simulink model "BD_SER2"  (Simulink 4.1.1)
settings: Solver=ode1  SolverMode=SingleTasking  StartTime=0.0  StopTime=max(cyc_mph(:,1))  FixedStep=1  MaxStep=1  RelTol=1e-3  AbsTol=1e-3
undefined symbols (not defined in the file): air_cp, amb_tmp, cyc_avg_time, cyc_cargo_mass, cyc_elevation_init, cyc_filter_bool, cyc_grade, cyc_mph, enable_stop, ess_cap_scale, ess_coulombic_eff, ess_init_soc, ess_max_ah_cap, ess_max_volts, ess_min_volts, ess_mod_airflow, ess_mod_cp, ess_mod_init_tmp, ess_module_mass, ess_module_num, ess_on, ess_res_scale_coef, ess_res_scale_fun, ess_set_tmp, ess_th_calc, ess_th_res_off, ess_th_res_on, ess_tmp, ess_voc, ex_calc, fc_ct_trq, fc_emis, fc_inertia, fc_map_spd, fc_max_trq, fc_spd_scale, fc_trq_scale, fd_inertia, fd_loss, fd_ratio, gb_dnshift_load, gb_dnshift_spd, gb_gears_num, gb_inertia, gb_num_init, gb_ratio, gb_shift_delay, gb_spd_scale, gb_trq_scale, gb_upshift_load, gb_upshift_spd, gc_inertia, gc_map_spd, gc_map_trq, gc_max_crrnt, gc_max_trq, gc_outpwr_map, gc_overtrq_factor, gc_spd_scale, gc_trq_scale ... (+37)
libraries: lib_wheel2 x12, lib_accessory2 x4, lib_controls2 x3, lib_etc x2, lib_help x2, lib_fuel_converter x2, lib_drive_cycle2 x1, lib_interactive x1, lib_drive_cycle x1, lib_exhaust x1, lib_fuel_converter3 x1
(part 3 of 15)

== system BD_SER2/ACC ELEC <acce>/ACC ELEC model and interface/electrical accessory model ==
  note: Backward-Forward Models
  "requested electrical Power, out to the driveline (W)" : Inport  Port=1  LatchInput=off
  achieved power in from power source (W) : Inport  Port=2  LatchInput=off
  Block NOTES : Subsystem
      settings: RTWFcnNameOpts=Auto  RTWFileNameOpts=Auto
      mask Display: disp('Block\nNOTES')
  backward model : Subsystem
      settings: RTWFcnNameOpts=Auto  RTWFileNameOpts=Auto
  electrical power logging : lib_accessory2/SubLibraries/electrical power logging  eff=acc_mech_eff
      link override enhancedToWorkspace1/To Workspace: VariableName=acce_elec_pwr_in_a  SampleTime=-1  SaveFormat=Array
  enhancedToWorkspace : Subsystem  TreatAsAtomicUnit=on  mask(enhancedToWorkspace){generalName=generalName, specificName=elec_pwr_a, logFlag=logFlag}
      mask prompts: generalName "General Name [char-evaluated]"; specificName "Specific Name [char-literal]"; logFlag "Enable flag (1=on,0=off)"
      mask help: A wrapper for the Simulink "To Workspace" block that allows you to evaluate the name of the variable to log to workspace. This is useful to avoid the double logging errors that occur when you pull in two library models that attempt to log to the same variable.
      mask init:
      | enhancedToWsMaker
      settings: CopyFcn=breakLinkCopyFcn  ParentCloseFcn=breakLinkParCloseFcn  RTWFcnNameOpts=Auto  RTWFileNameOpts=Auto
      mask Help:
      | <h2>Enhanced To Workspace Block</h2>
      | <h3>Parameters</h3>
      | <UL>
      | <li><b>General Name:</b> This is the more general name of the variable. Variables are saved to the workspace as <i>generalName_specificName</i>. Note that this is an evaluated variable. If you would like to type in the value directly, it must be surrounded with single quotes. Otherwise you can input the name of a variable containing a char string.</li>
      | <li><b>Specific Name:</b> This is the specific name of the variable. Note that this is input as a char literal (i.e., you don't need quotes).</li>
      | <li><b>Enable Flag:</b> This flag should have the value of 0 or 1. If 0, the variable will not be logged to the workspace. If 1, the variable will be logged. This is done so that variable logging can be turned off to improve speed.</li>
      | </ul>
      | <h3>Overview</h3>
      | <p>The enhanced to workspace block was put together to allow one to dynamically resolve variable names at run time in simulink. This is most powerful when used in conjunction with a masked subsystem to allow multiple instances of that masked subsytem to be used in the same model. The strategy is to set the generalName in the block mask which will allow the block to change the general name for all variable logging on the fly.
      | <h3>Helper Files</h3>
      | <p>Three m-files are required by the enhancedToWorkspace block. These files are located in the &lt; ADVISOR root &gt;/GUI directory :
      | <ul>
      | <li><i>enhancedToWsMaker.m</i> This file runs the mask initialization for the block</li>
      | <li><i>breakLinkCopyFcn.m</i> This file is used by the block callback when the simulink block is copied. It is necessary to break the link to the enhancedToWorkspace similar to the To Workspace block in order for it to be able to configure itself. (Try copying simulink's To Workspace block--it is impossible to make a link)</li>
      | <li><i>breakLinkParCloseFcn.m</i> This file is similar to the breakLinkCopyFcn and is used when a parent system is closed</li>
      | </ul>
      | <hr>
      | 
      | <p>Created 2003-Jan-21, Michael Patrick O'Keefe, NREL</p>
      | 
      | <!--
      | <VARDEF>
      | <H3>var_name</H3>
      | <UL>
      | <LI><B>data type</B> data type here</LI>
      | <LI><B>units</B> units here</LI>
      | <LI><B>vehicle type</B> vehicle type here</LI>
      | <LI><B>description</B> description here</LI>
      | </UL>
      | </VARDEF>
      | -->
      mask Display: disp([generalName,'_',specificName])
  enhancedToWorkspace1 : Subsystem  TreatAsAtomicUnit=on  mask(enhancedToWorkspace){generalName=generalName, specificName=elec_pwr_r, logFlag=logFlag}
      mask prompts: generalName "General Name [char-evaluated]"; specificName "Specific Name [char-literal]"; logFlag "Enable flag (1=on,0=off)"
      mask help: A wrapper for the Simulink "To Workspace" block that allows you to evaluate the name of the variable to log to workspace. This is useful to avoid the double logging errors that occur when you pull in two library models that attempt to log to the same variable.
      mask init:
      | enhancedToWsMaker
      settings: CopyFcn=breakLinkCopyFcn  ParentCloseFcn=breakLinkParCloseFcn  RTWFcnNameOpts=Auto  RTWFileNameOpts=Auto
      mask Help:
      | <h2>Enhanced To Workspace Block</h2>
      | <h3>Parameters</h3>
      | <UL>
      | <li><b>General Name:</b> This is the more general name of the variable. Variables are saved to the workspace as <i>generalName_specificName</i>. Note that this is an evaluated variable. If you would like to type in the value directly, it must be surrounded with single quotes. Otherwise you can input the name of a variable containing a char string.</li>
      | <li><b>Specific Name:</b> This is the specific name of the variable. Note that this is input as a char literal (i.e., you don't need quotes).</li>
      | <li><b>Enable Flag:</b> This flag should have the value of 0 or 1. If 0, the variable will not be logged to the workspace. If 1, the variable will be logged. This is done so that variable logging can be turned off to improve speed.</li>
      | </ul>
      | <h3>Overview</h3>
      | <p>The enhanced to workspace block was put together to allow one to dynamically resolve variable names at run time in simulink. This is most powerful when used in conjunction with a masked subsystem to allow multiple instances of that masked subsytem to be used in the same model. The strategy is to set the generalName in the block mask which will allow the block to change the general name for all variable logging on the fly.
      | <h3>Helper Files</h3>
      | <p>Three m-files are required by the enhancedToWorkspace block. These files are located in the &lt; ADVISOR root &gt;/GUI directory :
      | <ul>
      | <li><i>enhancedToWsMaker.m</i> This file runs the mask initialization for the block</li>
      | <li><i>breakLinkCopyFcn.m</i> This file is used by the block callback when the simulink block is copied. It is necessary to break the link to the enhancedToWorkspace similar to the To Workspace block in order for it to be able to configure itself. (Try copying simulink's To Workspace block--it is impossible to make a link)</li>
      | <li><i>breakLinkParCloseFcn.m</i> This file is similar to the breakLinkCopyFcn and is used when a parent system is closed</li>
      | </ul>
      | <hr>
      | 
      | <p>Created 2003-Jan-21, Michael Patrick O'Keefe, NREL</p>
      | 
      | <!--
      | <VARDEF>
      | <H3>var_name</H3>
      | <UL>
      | <LI><B>data type</B> data type here</LI>
      | <LI><B>units</B> units here</LI>
      | <LI><B>vehicle type</B> vehicle type here</LI>
      | <LI><B>description</B> description here</LI>
      | </UL>
      | </VARDEF>
      | -->
      mask Display: disp([generalName,'_',specificName])
  forward model : Subsystem
      settings: RTWFcnNameOpts=Auto  RTWFileNameOpts=Auto
  "requested electrical Power, in from the power source (W)" : Outport  Port=1
  "achieved electrical Power, out to the driveline (W)" : Outport  Port=2
  tag scope: acc_elec_pwr_a=scoped, acc_elec_pwr_r=scoped
  wires:
  forward model/2(acc_pwr_out) -> electrical power logging/1, enhancedToWorkspace/1(In1), [acc_elec_pwr_a]
  backward model/2(elec_acc_out) -> enhancedToWorkspace1/1(In1), forward model/2(acc_pwr_in), [acc_elec_pwr_r]
  forward model/1(pwr_out) -> "achieved electrical Power, out to the driveline (W)"/1
  achieved power in from power source (W)/1 -> forward model/1(pwr_in)
  backward model/1(elec_out) -> "requested electrical Power, in from the power source (W)"/1
  "requested electrical Power, out to the driveline (W)"/1 -> backward model/1(pwr_in)

== system BD_SER2/ACC ELEC <acce>/ACC ELEC model and interface/signal annotator ==
  In1 : Inport  Port=1  LatchInput=off
  Out1 : Outport  Port=1
  wires:
  In1/1 -> Out1/1  "driveline_elec_pwr_r"

== system BD_SER2/ACC MECH <accm>/mechanical accessory model and interface/Block NOTES ==

== system BD_SER2/ACC MECH <accm>/mechanical accessory model and interface/Mechanical Accessory model ==
  note: Reference Speed for speed dependant accessories
  note: Backward-Forward Models
  "requested shaft T and w, out to the driveline  (Nm ; rad/s; rad/s)" : Inport  Port=1  LatchInput=off
  "achieved shaft and belt T and w, in from the prime mover (Nm ; rad/s)" : Inport  Port=2  LatchInput=off
  Block NOTES : Subsystem
      settings: RTWFcnNameOpts=Auto  RTWFileNameOpts=Auto
      mask Display: disp('Block\nNOTES')
  Demux : Demux  Outputs=2  BusSelectionMode=off
  Demux1 : Demux  Outputs=2  BusSelectionMode=off
  Mux1 : Mux  Inputs=2
  Mux2 : Mux  Inputs=2
  backward model : Subsystem
      settings: RTWFcnNameOpts=Auto  RTWFileNameOpts=Auto
  f1 : Subsystem  TreatAsAtomicUnit=on  mask(enhancedToWorkspace){generalName=generalName, specificName=mech_pwr_a, logFlag=logFlag}
      mask prompts: generalName "General Name [char-evaluated]"; specificName "Specific Name [char-literal]"; logFlag "Enable flag (1=on,0=off)"
      mask help: A wrapper for the Simulink "To Workspace" block that allows you to evaluate the name of the variable to log to workspace. This is useful to avoid the double logging errors that occur when you pull in two library models that attempt to log to the same variable.
      mask init:
      | enhancedToWsMaker
      settings: CopyFcn=breakLinkCopyFcn  ParentCloseFcn=breakLinkParCloseFcn  RTWFcnNameOpts=Auto  RTWFileNameOpts=Auto
      mask Help:
      | <h2>Enhanced To Workspace Block</h2>
      | <h3>Parameters</h3>
      | <UL>
      | <li><b>General Name:</b> This is the more general name of the variable. Variables are saved to the workspace as <i>generalName_specificName</i>. Note that this is an evaluated variable. If you would like to type in the value directly, it must be surrounded with single quotes. Otherwise you can input the name of a variable containing a char string.</li>
      | <li><b>Specific Name:</b> This is the specific name of the variable. Note that this is input as a char literal (i.e., you don't need quotes).</li>
      | <li><b>Enable Flag:</b> This flag should have the value of 0 or 1. If 0, the variable will not be logged to the workspace. If 1, the variable will be logged. This is done so that variable logging can be turned off to improve speed.</li>
      | </ul>
      | <h3>Overview</h3>
      | <p>The enhanced to workspace block was put together to allow one to dynamically resolve variable names at run time in simulink. This is most powerful when used in conjunction with a masked subsystem to allow multiple instances of that masked subsytem to be used in the same model. The strategy is to set the generalName in the block mask which will allow the block to change the general name for all variable logging on the fly.
      | <h3>Helper Files</h3>
      | <p>Three m-files are required by the enhancedToWorkspace block. These files are located in the &lt; ADVISOR root &gt;/GUI directory :
      | <ul>
      | <li><i>enhancedToWsMaker.m</i> This file runs the mask initialization for the block</li>
      | <li><i>breakLinkCopyFcn.m</i> This file is used by the block callback when the simulink block is copied. It is necessary to break the link to the enhancedToWorkspace similar to the To Workspace block in order for it to be able to configure itself. (Try copying simulink's To Workspace block--it is impossible to make a link)</li>
      | <li><i>breakLinkParCloseFcn.m</i> This file is similar to the breakLinkCopyFcn and is used when a parent system is closed</li>
      | </ul>
      | <hr>
      | 
      | <p>Created 2003-Jan-21, Michael Patrick O'Keefe, NREL</p>
      | 
      | <!--
      | <VARDEF>
      | <H3>var_name</H3>
      | <UL>
      | <LI><B>data type</B> data type here</LI>
      | <LI><B>units</B> units here</LI>
      | <LI><B>vehicle type</B> vehicle type here</LI>
      | <LI><B>description</B> description here</LI>
      | </UL>
      | </VARDEF>
      | -->
      mask Display: disp([generalName,'_',specificName])
  f2 : Subsystem  TreatAsAtomicUnit=on  mask(enhancedToWorkspace){generalName=generalName, specificName=mech_trq_a, logFlag=logFlag}
      mask prompts: generalName "General Name [char-evaluated]"; specificName "Specific Name [char-literal]"; logFlag "Enable flag (1=on,0=off)"
      mask help: A wrapper for the Simulink "To Workspace" block that allows you to evaluate the name of the variable to log to workspace. This is useful to avoid the double logging errors that occur when you pull in two library models that attempt to log to the same variable.
      mask init:
      | enhancedToWsMaker
      settings: CopyFcn=breakLinkCopyFcn  ParentCloseFcn=breakLinkParCloseFcn  RTWFcnNameOpts=Auto  RTWFileNameOpts=Auto
      mask Help:
      | <h2>Enhanced To Workspace Block</h2>
      | <h3>Parameters</h3>
      | <UL>
      | <li><b>General Name:</b> This is the more general name of the variable. Variables are saved to the workspace as <i>generalName_specificName</i>. Note that this is an evaluated variable. If you would like to type in the value directly, it must be surrounded with single quotes. Otherwise you can input the name of a variable containing a char string.</li>
      | <li><b>Specific Name:</b> This is the specific name of the variable. Note that this is input as a char literal (i.e., you don't need quotes).</li>
      | <li><b>Enable Flag:</b> This flag should have the value of 0 or 1. If 0, the variable will not be logged to the workspace. If 1, the variable will be logged. This is done so that variable logging can be turned off to improve speed.</li>
      | </ul>
      | <h3>Overview</h3>
      | <p>The enhanced to workspace block was put together to allow one to dynamically resolve variable names at run time in simulink. This is most powerful when used in conjunction with a masked subsystem to allow multiple instances of that masked subsytem to be used in the same model. The strategy is to set the generalName in the block mask which will allow the block to change the general name for all variable logging on the fly.
      | <h3>Helper Files</h3>
      | <p>Three m-files are required by the enhancedToWorkspace block. These files are located in the &lt; ADVISOR root &gt;/GUI directory :
      | <ul>
      | <li><i>enhancedToWsMaker.m</i> This file runs the mask initialization for the block</li>
      | <li><i>breakLinkCopyFcn.m</i> This file is used by the block callback when the simulink block is copied. It is necessary to break the link to the enhancedToWorkspace similar to the To Workspace block in order for it to be able to configure itself. (Try copying simulink's To Workspace block--it is impossible to make a link)</li>
      | <li><i>breakLinkParCloseFcn.m</i> This file is similar to the breakLinkCopyFcn and is used when a parent system is closed</li>
      | </ul>
      | <hr>
      | 
      | <p>Created 2003-Jan-21, Michael Patrick O'Keefe, NREL</p>
      | 
      | <!--
      | <VARDEF>
      | <H3>var_name</H3>
      | <UL>
      | <LI><B>data type</B> data type here</LI>
      | <LI><B>units</B> units here</LI>
      | <LI><B>vehicle type</B> vehicle type here</LI>
      | <LI><B>description</B> description here</LI>
      | </UL>
      | </VARDEF>
      | -->
      mask Display: disp([generalName,'_',specificName])
  forward model : Subsystem
      settings: RTWFcnNameOpts=Auto  RTWFileNameOpts=Auto
  limit accessory mechanical speed achieved : lib_etc/saturation with inputs
      settings: RTWFcnNameOpts=Auto  RTWFileNameOpts=Auto
  limit accessory mechanical speed request : lib_etc/saturation with inputs
      settings: RTWFcnNameOpts=Auto  RTWFileNameOpts=Auto
  mechanical power logging : lib_accessory2/SubLibraries/mechanical power logging  eff=acc_mech_eff
  "requested shaft and belt T and w, in from the prime mover (Nm ; rad/s)" : Outport  Port=1
  "achieved shaft T and w, out to the driveline (Nm ; rad/s)" : Outport  Port=2
  tag scope: acc_mech_pwr_a=scoped, acc_mech_trq_a=scoped, w_APU_speed=scoped
  wires:
  [acc_min_spd] -> limit accessory mechanical speed achieved/3
  [acc_max_spd] -> limit accessory mechanical speed achieved/1
  [acc_mech_spd_a] -> limit accessory mechanical speed achieved/2
  limit accessory mechanical speed achieved/1 -> forward model/2(spd_in)
  [acc_min_spd] -> limit accessory mechanical speed request/3
  [acc_max_spd] -> limit accessory mechanical speed request/1
  limit accessory mechanical speed request/1 -> [w_APU_speed], backward model/2(spd_in)
  [acc_mech_spd_r] -> limit accessory mechanical speed request/2
  [acc_mech_trq_r] -> forward model/3(acc_trq_req)
  forward model/3(acc_mech_pwr_a) -> mechanical power logging/1, f1/1(In1), [acc_mech_pwr_a]
  forward model/2(acc_mech_trq_a) -> f2/1(In1), [acc_mech_trq_a]
  Mux2/1 -> "achieved shaft T and w, out to the driveline (Nm ; rad/s)"/1
  Mux1/1 -> "requested shaft and belt T and w, in from the prime mover (Nm ; rad/s)"/1
  "achieved shaft and belt T and w, in from the prime mover (Nm ; rad/s)"/1 -> Demux1/1
  "requested shaft T and w, out to the driveline  (Nm ; rad/s; rad/s)"/1 -> Demux/1
  Demux/1 -> backward model/1(trq1)  "trq out r"
  Demux/2 -> Mux1/2  "w shaft out r"
  backward model/1(trq2) -> Mux1/1  "trq in r"
  forward model/1(trq_out) -> Mux2/1
  Demux1/1 -> forward model/1(trq_in)  "trq in achieved from prime mover"
  Demux1/2 -> Mux2/2  "w shaft achieved by prime mover"

== system BD_SER2/ACC MECH <accm>/mechanical accessory model and interface/help ==

== system BD_SER2/ACC MECH <accm>/mechanical accessory model and interface/signal annotator ==
  In1 : Inport  Port=1  LatchInput=off
  Demux : Demux  Outputs=2  BusSelectionMode=off
  Mux : Mux  Inputs=2
  enhancedToWorkspace : Subsystem  TreatAsAtomicUnit=on  mask(enhancedToWorkspace){generalName=generalName, specificName=pre_acc_spd_out_r, logFlag=logFlag}
      mask prompts: generalName "General Name [char-evaluated]"; specificName "Specific Name [char-literal]"; logFlag "Enable flag (1=on,0=off)"
      mask help: A wrapper for the Simulink "To Workspace" block that allows you to evaluate the name of the variable to log to workspace. This is useful to avoid the double logging errors that occur when you pull in two library models that attempt to log to the same variable.
      mask init:
      | enhancedToWsMaker
      settings: CopyFcn=breakLinkCopyFcn  ParentCloseFcn=breakLinkParCloseFcn  RTWFcnNameOpts=Auto  RTWFileNameOpts=Auto
      mask Help:
      | <h2>Enhanced To Workspace Block</h2>
      | <h3>Parameters</h3>
      | <UL>
      | <li><b>General Name:</b> This is the more general name of the variable. Variables are saved to the workspace as <i>generalName_specificName</i>. Note that this is an evaluated variable. If you would like to type in the value directly, it must be surrounded with single quotes. Otherwise you can input the name of a variable containing a char string.</li>
      | <li><b>Specific Name:</b> This is the specific name of the variable. Note that this is input as a char literal (i.e., you don't need quotes).</li>
      | <li><b>Enable Flag:</b> This flag should have the value of 0 or 1. If 0, the variable will not be logged to the workspace. If 1, the variable will be logged. This is done so that variable logging can be turned off to improve speed.</li>
      | </ul>
      | <h3>Overview</h3>
      | <p>The enhanced to workspace block was put together to allow one to dynamically resolve variable names at run time in simulink. This is most powerful when used in conjunction with a masked subsystem to allow multiple instances of that masked subsytem to be used in the same model. The strategy is to set the generalName in the block mask which will allow the block to change the general name for all variable logging on the fly.
      | <h3>Helper Files</h3>
      | <p>Three m-files are required by the enhancedToWorkspace block. These files are located in the &lt; ADVISOR root &gt;/GUI directory :
      | <ul>
      | <li><i>enhancedToWsMaker.m</i> This file runs the mask initialization for the block</li>
      | <li><i>breakLinkCopyFcn.m</i> This file is used by the block callback when the simulink block is copied. It is necessary to break the link to the enhancedToWorkspace similar to the To Workspace block in order for it to be able to configure itself. (Try copying simulink's To Workspace block--it is impossible to make a link)</li>
      | <li><i>breakLinkParCloseFcn.m</i> This file is similar to the breakLinkCopyFcn and is used when a parent system is closed</li>
      | </ul>
      | <hr>
      | 
      | <p>Created 2003-Jan-21, Michael Patrick O'Keefe, NREL</p>
      | 
      | <!--
      | <VARDEF>
      | <H3>var_name</H3>
      | <UL>
      | <LI><B>data type</B> data type here</LI>
      | <LI><B>units</B> units here</LI>
      | <LI><B>vehicle type</B> vehicle type here</LI>
      | <LI><B>description</B> description here</LI>
      | </UL>
      | </VARDEF>
      | -->
      mask Display: disp([generalName,'_',specificName])
  enhancedToWorkspace1 : Subsystem  TreatAsAtomicUnit=on  mask(enhancedToWorkspace){generalName=generalName, specificName=pre_acc_trq_out_r, logFlag=logFlag}
      mask prompts: generalName "General Name [char-evaluated]"; specificName "Specific Name [char-literal]"; logFlag "Enable flag (1=on,0=off)"
      mask help: A wrapper for the Simulink "To Workspace" block that allows you to evaluate the name of the variable to log to workspace. This is useful to avoid the double logging errors that occur when you pull in two library models that attempt to log to the same variable.
      mask init:
      | enhancedToWsMaker
      settings: CopyFcn=breakLinkCopyFcn  ParentCloseFcn=breakLinkParCloseFcn  RTWFcnNameOpts=Auto  RTWFileNameOpts=Auto
      mask Help:
      | <h2>Enhanced To Workspace Block</h2>
      | <h3>Parameters</h3>
      | <UL>
      | <li><b>General Name:</b> This is the more general name of the variable. Variables are saved to the workspace as <i>generalName_specificName</i>. Note that this is an evaluated variable. If you would like to type in the value directly, it must be surrounded with single quotes. Otherwise you can input the name of a variable containing a char string.</li>
      | <li><b>Specific Name:</b> This is the specific name of the variable. Note that this is input as a char literal (i.e., you don't need quotes).</li>
      | <li><b>Enable Flag:</b> This flag should have the value of 0 or 1. If 0, the variable will not be logged to the workspace. If 1, the variable will be logged. This is done so that variable logging can be turned off to improve speed.</li>
      | </ul>
      | <h3>Overview</h3>
      | <p>The enhanced to workspace block was put together to allow one to dynamically resolve variable names at run time in simulink. This is most powerful when used in conjunction with a masked subsystem to allow multiple instances of that masked subsytem to be used in the same model. The strategy is to set the generalName in the block mask which will allow the block to change the general name for all variable logging on the fly.
      | <h3>Helper Files</h3>
      | <p>Three m-files are required by the enhancedToWorkspace block. These files are located in the &lt; ADVISOR root &gt;/GUI directory :
      | <ul>
      | <li><i>enhancedToWsMaker.m</i> This file runs the mask initialization for the block</li>
      | <li><i>breakLinkCopyFcn.m</i> This file is used by the block callback when the simulink block is copied. It is necessary to break the link to the enhancedToWorkspace similar to the To Workspace block in order for it to be able to configure itself. (Try copying simulink's To Workspace block--it is impossible to make a link)</li>
      | <li><i>breakLinkParCloseFcn.m</i> This file is similar to the breakLinkCopyFcn and is used when a parent system is closed</li>
      | </ul>
      | <hr>
      | 
      | <p>Created 2003-Jan-21, Michael Patrick O'Keefe, NREL</p>
      | 
      | <!--
      | <VARDEF>
      | <H3>var_name</H3>
      | <UL>
      | <LI><B>data type</B> data type here</LI>
      | <LI><B>units</B> units here</LI>
      | <LI><B>vehicle type</B> vehicle type here</LI>
      | <LI><B>description</B> description here</LI>
      | </UL>
      | </VARDEF>
      | -->
      mask Display: disp([generalName,'_',specificName])
  Out1 : Outport  Port=1
  wires:
  Mux/1 -> Out1/1
  Demux/2 -> Mux/2, enhancedToWorkspace/1(In1)  "macc_spd_out_r"
  Demux/1 -> Mux/1, enhancedToWorkspace1/1(In1)  "macc_trq_out_r"
  In1/1 -> Demux/1

== system BD_SER2/drive cycle <cyc>/drive cycle model and interface/drive cycle model ==
  Backlash : Backlash  BacklashWidth=0.5  InitialOutput=0
  Block NOTES : Subsystem
      settings: RTWFcnNameOpts=Auto  RTWFileNameOpts=Auto
      mask Display: disp('Block\nNOTES')
  Constant : Constant  Value=0.001
  Constant1 : Constant  Orientation=left  Value=0
  Constant2 : Constant  Value=cyc_filter_bool
  Derivative : Derivative
  Integrator : Integrator  ExternalReset=none  InitialConditionSource=internal  InitialCondition=cyc_elevation_init  LimitOutput=off  UpperSaturationLimit=inf  LowerSaturationLimit=-inf  ShowSaturationPort=off  ShowStatePort=off  AbsoluteTolerance=auto
  Product : Product  Inputs=2  Multiplication=Element-wise(.*)  SaturateOnIntegerOverflow=on
  Relational Operator : RelationalOperator  Operator=>
  Switch : Switch  Threshold=eps
  Switch1 : Switch  Threshold=eps
  Switch2 : Switch  Threshold=1
  Switch3 : Switch  Threshold=1
  Trigonometric Function : Trigonometry  Operator=sin  OutputSignalType=auto
  distance travelled (m) : Subsystem
      settings: RTWFcnNameOpts=Auto  RTWFileNameOpts=Auto
  enhancedToWorkspace : Subsystem  TreatAsAtomicUnit=on  mask(enhancedToWorkspace){generalName=generalName, specificName=cargo_mass_vs_time, logFlag=logFlag}
      mask prompts: generalName "General Name [char-evaluated]"; specificName "Specific Name [char-literal]"; logFlag "Enable flag (1=on,0=off)"
      mask help: A wrapper for the Simulink "To Workspace" block that allows you to evaluate the name of the variable to log to workspace. This is useful to avoid the double logging errors that occur when you pull in two library models that attempt to log to the same variable.
      mask init:
      | enhancedToWsMaker
      settings: CopyFcn=breakLinkCopyFcn  ParentCloseFcn=breakLinkParCloseFcn  RTWFcnNameOpts=Auto  RTWFileNameOpts=Auto
      mask Help:
      | <h2>Enhanced To Workspace Block</h2>
      | <h3>Parameters</h3>
      | <UL>
      | <li><b>General Name:</b> This is the more general name of the variable. Variables are saved to the workspace as <i>generalName_specificName</i>. Note that this is an evaluated variable. If you would like to type in the value directly, it must be surrounded with single quotes. Otherwise you can input the name of a variable containing a char string.</li>
      | <li><b>Specific Name:</b> This is the specific name of the variable. Note that this is input as a char literal (i.e., you don't need quotes).</li>
      | <li><b>Enable Flag:</b> This flag should have the value of 0 or 1. If 0, the variable will not be logged to the workspace. If 1, the variable will be logged. This is done so that variable logging can be turned off to improve speed.</li>
      | </ul>
      | <h3>Overview</h3>
      | <p>The enhanced to workspace block was put together to allow one to dynamically resolve variable names at run time in simulink. This is most powerful when used in conjunction with a masked subsystem to allow multiple instances of that masked subsytem to be used in the same model. The strategy is to set the generalName in the block mask which will allow the block to change the general name for all variable logging on the fly.
      | <h3>Helper Files</h3>
      | <p>Three m-files are required by the enhancedToWorkspace block. These files are located in the &lt; ADVISOR root &gt;/GUI directory :
      | <ul>
      | <li><i>enhancedToWsMaker.m</i> This file runs the mask initialization for the block</li>
      | <li><i>breakLinkCopyFcn.m</i> This file is used by the block callback when the simulink block is copied. It is necessary to break the link to the enhancedToWorkspace similar to the To Workspace block in order for it to be able to configure itself. (Try copying simulink's To Workspace block--it is impossible to make a link)</li>
      | <li><i>breakLinkParCloseFcn.m</i> This file is similar to the breakLinkCopyFcn and is used when a parent system is closed</li>
      | </ul>
      | <hr>
      | 
      | <p>Created 2003-Jan-21, Michael Patrick O'Keefe, NREL</p>
      | 
      | <!--
      | <VARDEF>
      | <H3>var_name</H3>
      | <UL>
      | <LI><B>data type</B> data type here</LI>
      | <LI><B>units</B> units here</LI>
      | <LI><B>vehicle type</B> vehicle type here</LI>
      | <LI><B>description</B> description here</LI>
      | </UL>
      | </VARDEF>
      | -->
      mask Display: disp([generalName,'_',specificName])
  mph-->m/s : Gain  Gain=0.447  Multiplication=Element-wise(K.*u)  SaturateOnIntegerOverflow=on
  repeated cycle grade vs. distance : Subsystem  mask(Repeating table){t=cyc_grade(:,1), y=cyc_grade(:,2)}
      mask prompts: t "Input values:"; y "Output values:"
      mask help:
      | Repeating table.
      | Enter values of input and output for first cycle.
      mask init:
      | period = max(@1);
      settings: RTWFcnNameOpts=Auto  RTWFileNameOpts=Auto
      mask Help: Repeats cycle given in table. Input values should be monotonically increasing.
  repeated cycle speed vs. time : Subsystem  mask(Repeating table){@1=cyc_mph(:,1), @2=cyc_mph(:,2)}
      mask prompts: @1 "Time values:"; @2 "Output values:"
      mask help:
      | Repeating table.
      | Enter values of time and output for first cycle.
      mask init:
      | period = max(@1); t = @1; y = @2;
      settings: RTWFcnNameOpts=Auto  RTWFileNameOpts=Auto
      mask Help: Repeats cycle given in table. Time values should be monotonically increasing.
  repeated cycle vehicle cargo mass vs. distance : lib_drive_cycle/drive cycle <cyc>/repeated cycle grade vs. distance  t=cyc_cargo_mass(:,1)  y=cyc_cargo_mass(:,2)
  "super-smooth, no-lag trace" : Subsystem  mask(Smooth Cycle){t=cyc_mph(:,1), y=cyc_mph(:,2), avgtime=cyc_avg_time}
      mask prompts: t "Time vector for trace (s):"; y "Speed vector for trace (km/hr):"; avgtime "Averaging time (s):"
      mask help: Smooth Cycle
      mask init:
      | period = max(@1);,
      settings: RTWFcnNameOpts=Auto  RTWFileNameOpts=Auto
      mask Display: disp('SMOOTH\nCYCLE')
  req'd vehicle speed (m/s) : Outport  Port=1  InitialOutput=0
  tag scope: cyc_mph_r=scoped, cyc_mph_r_orig=scoped, distance=scoped, elevation=scoped, grade=scoped, grade_orig=scoped, veh_cargo_mass=scoped
  wires:
  repeated cycle vehicle cargo mass vs. distance/1 -> enhancedToWorkspace/1(In1), [veh_cargo_mass]
  [Altia_Run] -> Switch3/2
  [altia_grade] -> Switch3/1
  [Altia_Run] -> Switch2/2
  [altia_cyc_mph_r] -> Switch2/1
  mph-->m/s/1 -> req'd vehicle speed (m/s)/1
  Switch2/1 -> mph-->m/s/1, [cyc_mph_r]
  Constant2/1 -> Switch1/2
  Constant1/1 -> Switch/3
  Relational Operator/1 -> Switch/2
  Backlash/1 -> Switch/1
  Constant/1 -> Relational Operator/2
  "super-smooth, no-lag trace"/1(out_1) -> Relational Operator/1, Backlash/1
  Switch/1 -> Switch1/1
  repeated cycle speed vs. time/1(out_1) -> Switch1/3
  Switch1/1 -> [cyc_mph_r_orig], Switch2/3
  Product/1 -> Integrator/1
  Derivative/1 -> Product/1
  Trigonometric Function/1 -> Product/2
  Integrator/1 -> [elevation]
  Switch3/1 -> [grade], Trigonometric Function/1
  distance travelled (m)/1(Out1) -> repeated cycle vehicle cargo mass vs. distance/1, [distance], Derivative/1, repeated cycle grade vs. distance/1(distance travelled (m))
  repeated cycle grade vs. distance/1(out_1) -> Switch3/3, [grade_orig]

== system BD_SER2/drive cycle <cyc>/drive cycle model and interface/signal annotator ==
  note: initial speed in m/s
  In1 : Inport  Port=1  LatchInput=off
  In2 : Inport  Port=2  LatchInput=off
  In3 : Inport  Port=3  LatchInput=off
  Bus Creator : BusCreator  Inputs=4
  Constant : Constant  Value=cyc_mph(1,2)*.447
  Out1 : Outport  Port=1
  wires:
  Constant/1 -> Bus Creator/4  "v_init"
  In3/1 -> Bus Creator/3  "cycle_mph_r"
  In2/1 -> Bus Creator/2  "cycle_mph_r_orig"
  Bus Creator/1 -> Out1/1
  In1/1 -> Bus Creator/1  "simulation_time"

== system BD_SER2/ess config/energy storage <ess>/Block NOTES ==
  note: This is a stand-alone version of an energy storage system
      |
      | Several different models are available

== system BD_SER2/ess config/energy storage <ess>/documentation9 ==

== system BD_SER2/ess config/energy storage <ess>/energy storage <ess> ==
  note: Model
  note: Interface
  power req'd into bus (W) : Inport  Port=1  LatchInput=off
  control : Inport  Port=2  LatchInput=off
  Bus Creator : BusCreator  Inputs=12
  Goto Tag Visibility : GotoTagVisibility  GotoTag=ess_tmp
  Goto Tag Visibility1 : GotoTagVisibility  GotoTag=bus_voltage
  Goto Tag Visibility10 : GotoTagVisibility  GotoTag=mc_voltage_limited
  Goto Tag Visibility11 : GotoTagVisibility  GotoTag=ess_pwr_limited
  Goto Tag Visibility12 : GotoTagVisibility  GotoTag=ess_minV_limited
  Goto Tag Visibility2 : GotoTagVisibility  GotoTag=ess_max_pwr
  Goto Tag Visibility3 : GotoTagVisibility  GotoTag=ess_max_chg_pwr
  Goto Tag Visibility4 : GotoTagVisibility  GotoTag=ess_pwr_out_a
  Goto Tag Visibility6 : GotoTagVisibility  GotoTag=SOC
  Goto Tag Visibility7 : GotoTagVisibility  GotoTag=ess_maxV_limited
  Goto Tag Visibility8 : GotoTagVisibility  GotoTag=ess_soc_hi_limited
  Goto Tag Visibility9 : GotoTagVisibility  GotoTag=ess_soc_low_limited
  Model : Subsystem
      settings: RTWFcnNameOpts=Auto  RTWFileNameOpts=Auto
  Terminator : Terminator
  signal annotator : Subsystem
      settings: RTWFcnNameOpts=Auto  RTWFileNameOpts=Auto
  required out : Outport  Port=1  InitialOutput=0
  power available to bus (W) : Outport  Port=2  InitialOutput=0
  sensors : Outport  Port=3  InitialOutput=0
  wires:
  signal annotator/1(Out1) -> required out/1
  [ess_minV_limited] -> Bus Creator/12  "ess_minV_limited"
  [ess_pwr_limited] -> Bus Creator/11  "ess_pwr_limited"
  [mc_voltage_limited] -> Bus Creator/10  "mc_voltage_limited"
  [ess_soc_low_limited] -> Bus Creator/9  "ess_soc_low_limited"
  [ess_soc_hi_limited] -> Bus Creator/8  "ess_soc_hi_limited"
  [ess_maxV_limited] -> Bus Creator/7  "ess_maxV_limited"
  [SOC] -> Bus Creator/6  "SOC"
  [ess_max_pwr] -> Bus Creator/5  "ess_max_pwr"
  [ess_max_chg_pwr] -> Bus Creator/4  "ess_max_chg_pwr"
  [ess_pwr_out_a] -> Bus Creator/3  "ess_pwr_out_a"
  [bus_voltage] -> Bus Creator/2  "bus_voltage"
  Bus Creator/1 -> sensors/1
  control/1 -> Terminator/1
  [ess_tmp] -> Bus Creator/1  "ess_tmp"
  Model/1(power available to bus (W)) -> power available to bus (W)/1
  power req'd into bus (W)/1 -> signal annotator/1(In1), Model/1(power req'd into bus (W))
